simulink library "lib_Convection_TurbAxiSymAmbrok"  (R2015a)
settings: Solver=ode45  StartTime=0.0  StopTime=10.0  RelTol=1e-3
settings Model: Creator=jlkratz  LastModifiedBy=jlkratz

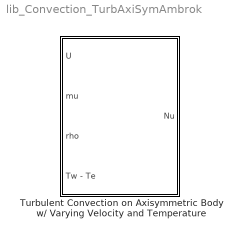
== system lib_Convection_TurbAxiSymAmbrok ==
  Turbulent Convection on Axisymmetric Body w/ Varying Velocity and Temperature : Subsystem  mask(Turbulent Convection on Axisymmetric Body w/ Varying Velocity and Temperature){Pr_M=1, x_M=[0.05:0.05:3], r0_M=linspace(0.01,1,60), BN_M=double(gcb)}
      mask prompts: Pr_M "Pr_M - Prandtl number [1x1]"; x_M "x_M - Local axial position [nx1]"; r0_M "r0_M - Local radius of the axisymmetric body [nx1]"; BN_M "BN_M -Block name"
      mask help:
      | This block implements a simple and reliable theory developed by Ambrok (1957) allows for the appsoximation of the local Stanton number of turbulent flow with a varying velocity and temperature profile along an axisymmetric body. When te radius, r0(x), is constant the Stanton number should give a descent approximation for a 2-D body. Ambrok's Stanton number correlation comes from solving a modeled energy-integral equation so that the local Stanton number could be approximated by simple quadrature. The Stanton number is then used to obtain the local Nusselt number.
      |
      | See the block help menu for more details.
      mask init:
      | %Error/Warning Checking --------------------------------------------------%
      | 
      | %---- Pr_M ----%
      | %Scalar?
      | if isscalar(Pr_M) == 0
      |     Pr_M = 1;
      |     fprintf('Warning in %s: Pr_M must be a scalar. Pr_M has been set equal to 1 for computations.\n',char(BN_M));
      | end
      | %Real?
      | if isreal(Pr_M) == 0
      |     Pr_M = real(Pr_M);
      |     fprintf('Warning in %s: Pr_M must be a real. Pr_M has been set equal to real part of the entered value for computations.\n',char(BN_M));
      | end
      | %Finite?
      | if isfinite(Pr_M) == 0
      |     Pr_M = 1;
      |     fprintf('Warning in %s: Pr_M must be a finite. Pr_M has been set equal to 1 for computations.\n',char(BN_M));
      | end
      | %greater than 0
      | if Pr_M <= 0
      |     Pr_M = 1;
      |     fprintf('Warning in %s: Pr_M must be positive. Pr_M has been set equal to 1 for computations.\n',char(BN_M));
      | end
      | %---- x_M ----%
      | %Not empty?
      | if isempty(x_M) == 1
      |     fprintf('Warning in %s: x_M cannot be empty.\n',char(BN_M));
      | end
      | %1-D array with 2 or more elements?
      | if min(size(x_M)) ~= 1 || length(size(x_M)) > 2 || max(size(x_M)) < 2
      |     fprintf('Warning in %s: x_M must be a 1-D array with at least 2 elements.\n',char(BN_M));
      | end
      | %Real?
      | if min(isreal(x_M)) == 0
      |     x_M = real(x_M);
      |     fprintf('Warning in %s: x_M must have all real elements. x_M has been set equal to the real parts of the entered values for computations.\n',char(BN_M));
      | end
      | %Finite?
      | if min(isfinite(x_M)) == 0
      |     fprintf('Warning in %s: x_M must have all finite elements.\n',char(BN_M));
      | end
      | %Greater than 0?
      | if min(x_M) <= 0
      |     fprintf('Warning in %s: x_M must have all elements that are greater than 0.\n',char(BN_M));
      | end
      | %Monotonically Increasing?
      | if max(size(x_M)) > 1
      |     if min(diff(x_M)) <= 0
      |         fprintf('Warning in %s: x_M must be a monotonically increasing array.\n',char(BN_M));
      |     end
      | end
      | %---- r0_M ----%
      | %Not empty?
      | if isempty(r0_M) == 1
      |     r0_M = ones(1,length(x_M));
      |     fprintf('Warning in %s: r0_M cannot be empty. r0_M has been set to a 1D array of ones the length of x_M for computations.\n',char(BN_M));
      | end
      | %1-D array?
      | if min(size(r0_M)) ~= 1 || length(size(r0_M)) > 2
      |     r0_M = ones(1,length(x_M));
      |     fprintf('Warning in %s: r0_M must be a 1-D array. r0_M has been set to a 1D array of ones the length of x_M for computations.\n',char(BN_M));
      | end
      | %Real?
      | if min(isreal(r0_M)) == 0
      |     r0_M = real(r0_M);
      |     fprintf('Warning in %s: r0_M must have all real elements. r0_M has been set equal to the real parts of the entered values for computations.\n',char(BN_M));
      | end
      | %Finite?
      | if min(isfinite(r0_M)) == 0
      |     r0_M = ones(1,length(x_M));
      |     fprintf('Warning in %s: r0_M must have all finite elements. r0_M has been set equal to a 1D array of ones the length of x_M for computations.\n',char(BN_M));
      | end
      | %Greater than 0?
      | if min(r0_M) <= 0
      |     r0_M = ones(1,length(x_M));
      |     fprintf('Warning in %s: r0_M must have all elements that are greater than 0. r0_M has been set equal to a 1D array of ones the length of x_M for computations.\n',char(BN_M));
      | end
      mask Help: web(which('Convection_TSAT_TurbAxisymBodyAmbrok.html'),'-helpbrowser')

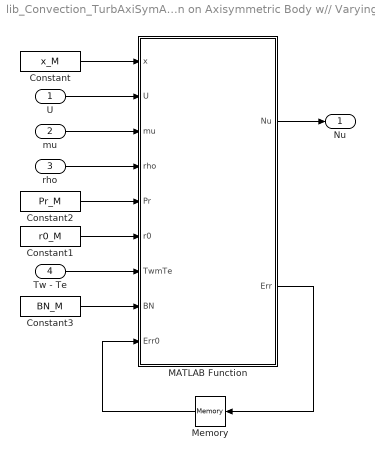
== system lib_Convection_TurbAxiSymAmbrok/Turbulent Convection on Axisymmetric Body w// Varying Velocity and Temperature ==
  U : Inport
  mu : Inport  Port=2
  rho : Inport  Port=3
  Tw - Te : Inport  Port=4
  Constant : Constant  Value=x_M
  Constant1 : Constant  Value=r0_M
  Constant2 : Constant  Value=Pr_M
  Constant3 : Constant  Value=BN_M
  MATLAB Function : MATLAB Function  TreatAsAtomicUnit=on
  Memory : Memory  X0=zeros(1,24)
  Nu : Outport
  wires:
  rho/1 -> MATLAB Function/4(rho)
  mu/1 -> MATLAB Function/3(mu)
  Constant1/1 -> MATLAB Function/6(r0)
  U/1 -> MATLAB Function/2(U)
  MATLAB Function/1(Nu) -> Nu/1
  Tw - Te/1 -> MATLAB Function/7(TwmTe)
  Constant2/1 -> MATLAB Function/5(Pr)
  Constant/1 -> MATLAB Function/1(x)
  Constant3/1 -> MATLAB Function/8(BN)
  MATLAB Function/2(Err) -> Memory/1
  Memory/1 -> MATLAB Function/9(Err0)

== matlab function lib_Convection_TurbAxiSymAmbrok/Turbulent Convection on Axisymmetric Body w// Varying Velocity and Temperature/MATLAB Function ==
  data: x input; Nu output; U input; mu input; rho input; Pr input; r0 input; TwmTe input; BN input; Err0 input; Err output
function [Nu,Err] = TurbFlwAxialBody(x,U,mu,rho,Pr,r0,TwmTe,BN,Err0)
%#codegen

%Error/Warning Checks ----------------------------------------------------%

Err = Err0;
ErrNum = 1;
%---- x and r0 ----%
%x and r0 are the same length
if length(x) ~= length(r0) && Err(ErrNum) < 1
    Err(ErrNum) = 1;
    fprintf('Warning in %s: x_M and r0_M should be the same length.\n',char(BN));
end
ErrNum = ErrNum + 1;
%---- U ----%
%Not empty?
if isempty(U) == 1 &&  Err(ErrNum) == 0
    Err(ErrNum) = 1;
    fprintf('Warning in %s: U is an empty array.\n',char(BN));
end
ErrNum = ErrNum + 1;
%1D array?
if (min(size(U)) > 1 || length(size(U)) > 2) && Err(ErrNum) == 0
    Err(ErrNum) = 1;
    fprintf('Warning in %s: U must be a 1-D array.\n',char(BN));
end
ErrNum = ErrNum + 1;
%Length of x?
if length(U) ~= length(x) && Err(ErrNum) == 0
    Err(ErrNum) = 1;
    fprintf('Warning in %s: U must have the same number of elements as x',char(BN));
end
ErrNum = ErrNum + 1;
%Real?
if min(isreal(U)) < 1 && Err(ErrNum) == 0
    Err(ErrNum) = 1;
    fprintf('Warning in %s: U must have all real elements.\n',char(BN));
end
ErrNum = ErrNum + 1;
%Finite?
if min(isfinite(U)) < 1 && Err(ErrNum) == 0
    Err(ErrNum) = 1;
    fprintf('Warning in %s: U must have all finite elements.\n',char(BN));
end
ErrNum = ErrNum + 1;
%Positive?
if min(U) <= 0 && Err(ErrNum) == 0
    Err(ErrNum) = 1;
    fprintf('Warning in %s: U must be great than 0.\n',char(BN));
end
ErrNum = ErrNum + 1;
%---- mu ----%
%Not empty?
if isempty(mu) == 1 &&  Err(ErrNum) == 0
    Err(ErrNum) = 1;
    fprintf('Warning in %s: mu is an empty array.\n',char(BN));
end
ErrNum = ErrNum + 1;
%1D array?
if (min(size(mu)) > 1 || length(size(mu)) > 2) && Err(ErrNum) == 0
    Err(ErrNum) = 1;
    fprintf('Warning in %s: mu must be a 1-D array.\n',char(BN));
end
ErrNum = ErrNum + 1;
%Length of x?
if length(mu) ~= length(x) && Err(ErrNum) == 0
    Err(ErrNum) = 1;
    fprintf('Warning in %s: mu must have the same number of elements as x',char(BN));
end
ErrNum = ErrNum + 1;
%Real?
if min(isreal(mu)) < 1 && Err(ErrNum) == 0
    Err(ErrNum) = 1;
    fprintf('Warning in %s: mu must have all real elements.\n',char(BN));
end
ErrNum = ErrNum + 1;
%Finite?
if min(isfinite(mu)) < 1 && Err(ErrNum) == 0
    Err(ErrNum) = 1;
    fprintf('Warning in %s: mu must have all finite elements.\n',char(BN));
end
ErrNum = ErrNum + 1;
%Positive?
if min(mu) <= 0 && Err(ErrNum) == 0
    Err(ErrNum) = 1;
    fprintf('Warning in %s: mu must be greater than 0.\n',char(BN));
end
ErrNum = ErrNum + 1;
%---- rho ----%
%Not empty?
if isempty(rho) == 1 &&  Err(ErrNum) == 0
    Err(ErrNum) = 1;
    fprintf('Warning in %s: rho is an empty array.\n',char(BN));
end
ErrNum = ErrNum + 1;
%1D array?
if (min(size(rho)) > 1 || length(size(rho)) > 2) && Err(ErrNum) == 0
    Err(ErrNum) = 1;
    fprintf('Warning in %s: rho must be a 1-D array.\n',char(BN));
end
ErrNum = ErrNum + 1;
%Length of x?
if length(rho) ~= length(x) && Err(ErrNum) == 0
    Err(ErrNum) = 1;
    fprintf('Warning in %s: rho must have the same number of elements as x',char(BN));
end
ErrNum = ErrNum + 1;
%Real?
if min(isreal(rho)) < 1 && Err(ErrNum) == 0
    Err(ErrNum) = 1;
    fprintf('Warning in %s: rho must have all real elements.\n',char(BN));
end
ErrNum = ErrNum + 1;
%Finite?
if min(isfinite(rho)) < 1 && Err(ErrNum) == 0
    Err(ErrNum) = 1;
    fprintf('Warning in %s: rho must have all finite elements.\n',char(BN));
end
ErrNum = ErrNum + 1;
%Positive?
if min(rho) <= 0 && Err(ErrNum) == 0
    Err(ErrNum) = 1;
    fprintf('Warning in %s: rho must be greater than 0.\n',char(BN));
end
ErrNum = ErrNum + 1;
%---- TwmTe ----%
if isempty(TwmTe) == 1 &&  Err(ErrNum) == 0
    Err(ErrNum) = 1;
    fprintf('Warning in %s: TwmTe is an empty array.\n',char(BN));
end
ErrNum = ErrNum + 1;
%1D array?
if (min(size(TwmTe)) > 1 || length(size(TwmTe)) > 2) && Err(ErrNum) == 0
    Err(ErrNum) = 1;
    fprintf('Warning in %s: TwmTe must be a 1-D array.\n',char(BN));
end
ErrNum = ErrNum + 1;
%Length of x?
if length(TwmTe) ~= length(x) && Err(ErrNum) == 0
    Err(ErrNum) = 1;
    fprintf('Warning in %s: TwmTe must have the same number of elements as x',char(BN));
end
ErrNum = ErrNum + 1;
%Real?
if min(isreal(TwmTe)) < 1 && Err(ErrNum) == 0
    Err(ErrNum) = 1;
    fprintf('Warning in %s: TwmTe must have all real elements.\n',char(BN));
end
ErrNum = ErrNum + 1;
%Finite?
if min(isfinite(TwmTe)) < 1 && Err(ErrNum) == 0
    Err(ErrNum) = 1;
    fprintf('Warning in %s: TwmTe must have all finite elements.\n',char(BN));
end

%Computations ------------------------------------------------------------%

NUM = zeros(1,length(x));
DEN = zeros(1,length(x));
INT = zeros(1,length(x)+1);
Nu = zeros(1,length(x));

Re = rho.*x.*U./mu;

INT(1) = 0;
for i = 1:length(x)
    NUM(i) = (r0(i)^0.25) * ((TwmTe(i))^(0.25)) * mu(i)^(0.2);
    INT(i+1) = (r0(i)^1.25) * ((TwmTe(i))^(1.25)) * (rho(i) * U(i));
end 
for i = 1:length(x);
    DEN(i) = trapz([0 x(1:i)'],INT(1:i+1))^(0.2);
end
St = 0.0295*Pr^(-0.4)*NUM./DEN;
for i = 1:length(x)
    Nu(i) = St(i)*Re(i)*Pr;
end
